simulink subsystem "HallSensor"  (R2022b)
settings: Solver=VariableStepAuto  StartTime=0.0  StopTime=10.0  RelTol=1e-3
undefined symbols (not defined in the file): ProjectExample
settings Model: Creator=Ilya_Andriyanov  LastModifiedBy=user

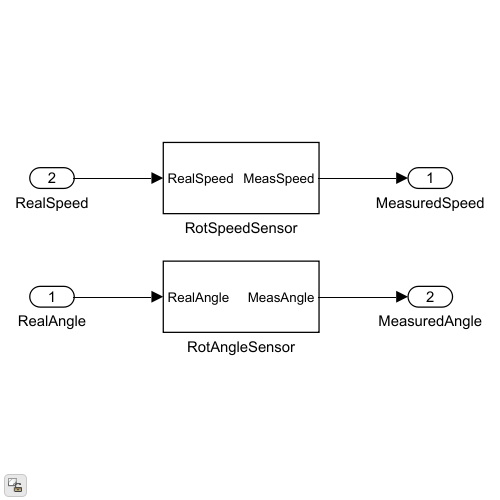
[thumbnail: Simulink's stored preview of the top-level diagram]
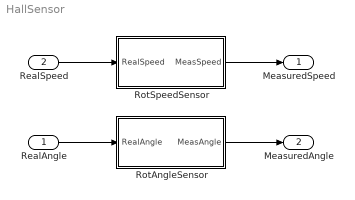
== system HallSensor ==
  RealAngle : Inport
  RealSpeed : Inport  Port=2
  RotAngleSensor : Subsystem
  RotSpeedSensor : Subsystem
  MeasuredSpeed : Outport
  MeasuredAngle : Outport  Port=2
  wires:
  RotSpeedSensor/1(MeasSpeed) -> MeasuredSpeed/1
  RealSpeed/1 -> RotSpeedSensor/1(RealSpeed)
  RotAngleSensor/1(MeasAngle) -> MeasuredAngle/1
  RealAngle/1 -> RotAngleSensor/1(RealAngle)

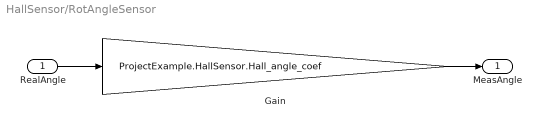
== system HallSensor/RotAngleSensor ==
  RealAngle : Inport
  Gain : Gain  Gain=ProjectExample.HallSensor.Hall_angle_coef
  MeasAngle : Outport
  wires:
  Gain/1 -> MeasAngle/1
  RealAngle/1 -> Gain/1

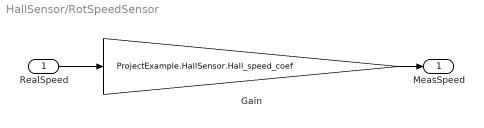
== system HallSensor/RotSpeedSensor ==
  RealSpeed : Inport
  Gain : Gain  Gain=ProjectExample.HallSensor.Hall_speed_coef
  MeasSpeed : Outport
  wires:
  Gain/1 -> MeasSpeed/1
  RealSpeed/1 -> Gain/1
